simulink model "A5_3_Sim_Lead_Continuous_Discrete_Comparison"  (Simulink 7.4)
settings: Solver=ode45  StartTime=0.0  StopTime=5  MaxStep=1e-3  RelTol=1e-3
settings Model: Creator=Natalia  LastModifiedBy=ma
settings DebuggingCC: StrictBusMsg=ErrorLevel1
settings HardwareCC: ProdIntDivRoundTo=Zero  ProdEndianess=LittleEndian  ProdHWDeviceType=Generic->32-bit x86 compatible
settings RTWCC: SystemTargetFile=rtwin.tlc  TemplateMakefile=rtwin.tmf  Description=Real-Time Windows Target  ProcessScript=rtwin_make_rtw_hook  RTWCompilerOptimization=On
settings CodeAppCC: MaxIdLength=95  CustomSymbolStrType=$N$R$M_T
settings TargetCC: TargetLibSuffix=_rtwin.lib  TargetPreCompLibLocation=C:\Program Files\MATLAB\R2012b\toolbox\rtw\targets\rtwin\lib\win64  TargetFunctionLibrary=ANSI_C  IsPILTarget=off  MatFileLogging=on  EnableShiftOperators=on
settings CustomProperty: DataType=string  Value=C:/PROGRA~1/MATLAB/R2012b/toolbox/rtw/targets/rtwin

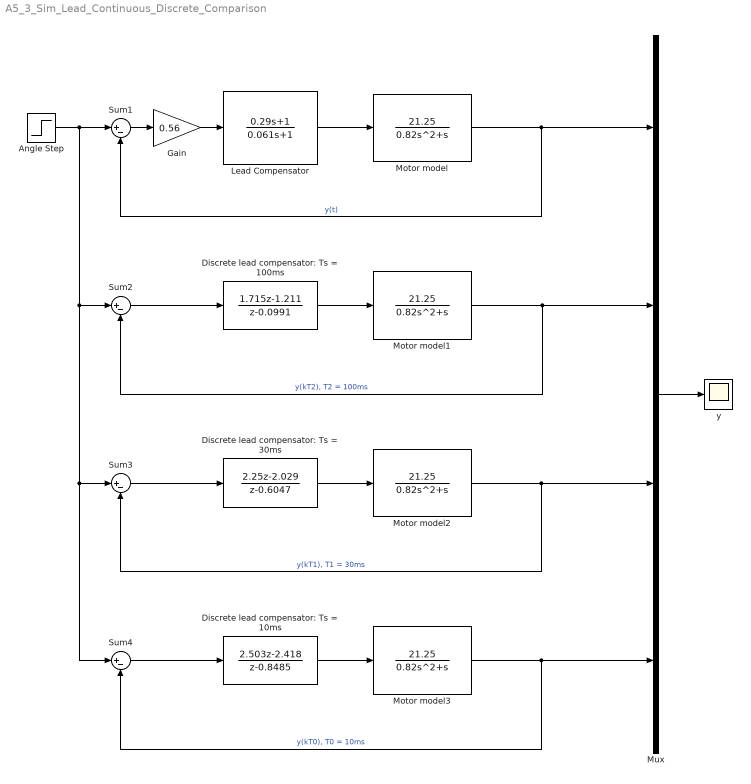
== system A5_3_Sim_Lead_Continuous_Discrete_Comparison ==
  Angle Step : Step  After=10  SampleTime=0
  Discrete lead compensator: Ts = 100ms : DiscreteTransferFcn  Numerator=[1.715 -1.211]  Denominator=[1 -0.0991]  SampleTime=0.1
  Discrete lead compensator: Ts = 10ms : DiscreteTransferFcn  Numerator=[2.503 -2.418]  Denominator=[1 -0.8485]  SampleTime=0.01
  Discrete lead compensator: Ts = 30ms : DiscreteTransferFcn  Numerator=[2.25 -2.029]  Denominator=[1 -0.6047]  SampleTime=0.03
  Gain : Gain  Gain=0.56
  Lead Compensator : TransferFcn  Numerator=[0.29 1]  Denominator=[0.061 1]
  Motor model{,1..3} (4 alike) : TransferFcn  Numerator=[21.25]  Denominator=[0.82 1 0]
  Mux : Mux
  Sum{1..4} (4 alike) : Sum  Inputs=|+-
  y : Scope
      settings: YMin=-0.5  YMax=11
  wires:
  Sum1/1 -> Gain/1
  Lead Compensator/1 -> Motor model/1
  Motor model/1 -> Sum1/2, Mux/1  "y(t)"
  Gain/1 -> Lead Compensator/1
  Sum2/1 -> Discrete lead compensator: Ts = 100ms/1
  Discrete lead compensator: Ts = 100ms/1 -> Motor model1/1
  Motor model1/1 -> Sum2/2, Mux/2  "y(kT2), T2 = 100ms"
  Sum3/1 -> Discrete lead compensator: Ts = 30ms/1
  Discrete lead compensator: Ts = 30ms/1 -> Motor model2/1
  Motor model2/1 -> Mux/3, Sum3/2  "y(kT1), T1 = 30ms"
  Angle Step/1 -> Sum2/1, Sum4/1, Sum3/1, Sum1/1
  Sum4/1 -> Discrete lead compensator: Ts = 10ms/1
  Discrete lead compensator: Ts = 10ms/1 -> Motor model3/1
  Motor model3/1 -> Mux/4, Sum4/2  "y(kT0), T0 = 10ms"
  Mux/1 -> y/1
